simulink model "etc"  (R2022b)
settings: Solver=ode45  StartTime=0.0  StopTime=10.0  RelTol=1e-3  EnableMultiTasking=on
PreLoadFcn:
  | load busData;
  | load globData;
undefined symbols (not defined in the file): digital_range, direction_range_analog, duty_range_analog, Ts, uint_range_10bit
libraries: adcUtils x2, SignalEditorBlockLib x2
settings Model: Creator=jrivitus  LastModifiedBy=bensweet
settings SolverCC: MaxConsecutiveZCs=25  AlgebraicLoopSolver=TrustRegion
settings DataIOCC: LimitDataPoints=on  SaveFormat=Array  SaveOutput=off  SaveTime=off  ReturnWorkspaceOutputs=off
settings OptimizationCC: DefaultParameterBehavior=Inlined  ExpressionDepthLimit=2147483647  InitFltsAndDblsToZero=on  LifeSpan=inf
settings DebuggingCC: SolverPrmCheckMsg=warning  ParameterPrecisionLossMsg=none  FcnCallInpInsideContextMsg=warning  UnconnectedInputMsg=warning  UnconnectedOutputMsg=warning  UnconnectedLineMsg=warning  StateNameClashWarn=warning  PregeneratedLibrarySubsystemCodeDiagnostic=none  SFUnexpectedBacktrackingDiag=warning  SFNoUnconditionalDefaultTransitionDiag=warning  SFExecutionAtInitializationDiag=none  SFMachineParentedDataDiag=warning  ArithmeticOperatorsInVariantConditions=warning
settings HardwareCC: ProdBitPerPointer=32  ProdBitPerSizeT=32  ProdBitPerPtrDiffT=32  ProdLargestAtomicFloat=None  ProdIntDivRoundTo=Undefined  ProdEndianess=Unspecified  ProdWordSize=32  ProdHWDeviceType=32-bit Generic
settings ModelReferenceCC: EnableRefExpFcnMdlSchedulingChecks=on  PropagateSignalLabelsOutOfModel=off
settings SFSimCC: SimUseLocalCustomCode=off
settings RTWCC: RTWUseLocalCustomCode=off  DLArmComputeVersion=19.05
settings CodeAppCC: StateflowObjectComments=on
settings GRTTargetCC: TargetLangStandard=C89/C90 (ANSI)  CombineOutputUpdateFcns=off  GRTInterface=on
settings ConfigComp: CovMetricSettings=dw  CovSaveCumulativeToWorkspaceVar=on  CovSaveSingleToWorkspaceVar=on  CovExternalEMLEnable=off  CovSFcnEnable=off

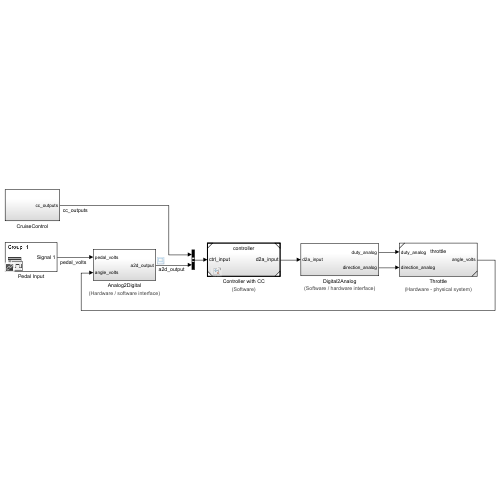
[thumbnail: Simulink's stored preview of the top-level diagram]
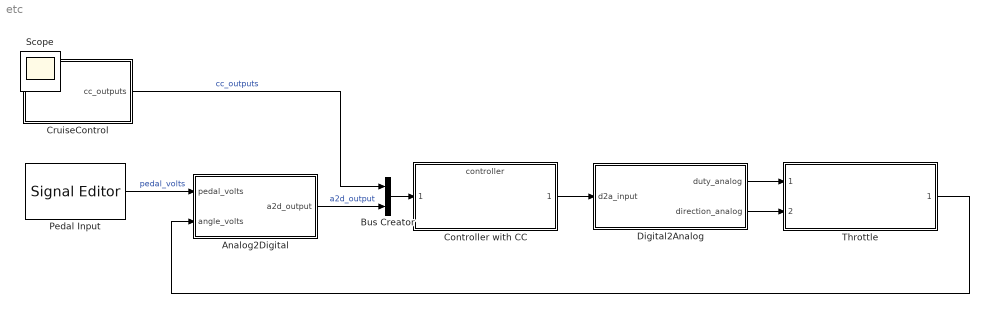
== system etc ==
  Analog2Digital : Subsystem
      settings: AttributesFormatString=(Hardware / software interface)  MinAlgLoopOccurrences=on
  Bus Creator : BusCreator  Inputs=2  OutDataTypeStr=Bus: ctrl_input_bus
  Controller with CC : ModelReference  ModelNameDialog=controller  SimulationMode=Normal  ModelReferenceVersion=6.0
      settings: AttributesFormatString=(Software)
  CruiseControl : Subsystem
      settings: MinAlgLoopOccurrences=on
  Digital2Analog : Subsystem
      settings: AttributesFormatString=(Software / hardware interface)  MinAlgLoopOccurrences=on
  Pedal Input : SignalEditorBlockLib/Signal Editor  FileName=etc_Pedal_Input.mat  ActiveScenario=Group_1  ActiveSignal=Signal 1  IsBus=off  OutputBusObjectStr=Bus: BusObject  SampleTime=0  OutputAfterFinalValue=Extrapolation  Unit=inherit  PreserveSignalName=on
  Throttle : Subsystem  ReferencedSubsystem=throttle
      settings: AttributesFormatString=(Hardware - physical system)
  Scope : Scope
  wires:
  Analog2Digital/1(a2d_output) -> Bus Creator/2  "a2d_output"
  CruiseControl/1(cc_outputs) -> Bus Creator/1  "cc_outputs"
  Digital2Analog/1(duty_analog) -> Throttle/1
  Digital2Analog/2(direction_analog) -> Throttle/2
  Throttle/1 -> Analog2Digital/2(angle_volts)
  Pedal Input/1 -> Analog2Digital/1(pedal_volts)  "pedal_volts"
  Bus Creator/1 -> Controller with CC/1
  Controller with CC/1 -> Digital2Analog/1(d2a_input)

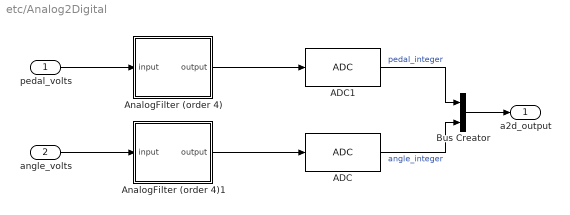
== system etc/Analog2Digital ==
  pedal_volts : Inport  OutDataTypeStr=double  PortDimensions=1  SampleTime=0
  angle_volts : Inport  Port=2  OutDataTypeStr=double  PortDimensions=1  SampleTime=0
  ADC : adcUtils/ADC  analog_range=angle_sensor_range  digital_range=uint_range_10bit  outputType=uint16  sampleTime=Ts
  ADC1 : adcUtils/ADC  analog_range=pedal_sensor_range  digital_range=uint_range_10bit  outputType=uint16  sampleTime=Ts
  AnalogFilter (order 4) : Subsystem  VariantControl=analogFilter==1
  AnalogFilter (order 4)1 : Subsystem  VariantControl=analogFilter==1
  Bus Creator : BusCreator  Inputs=2  OutDataTypeStr=Bus: a2d_output_bus
  a2d_output : Outport  OutDataTypeStr=Bus: a2d_output_bus  SampleTime=Ts  VectorParamsAs1DForOutWhenUnconnected=off
  wires:
  pedal_volts/1 -> AnalogFilter (order 4)/1(input)
  angle_volts/1 -> AnalogFilter (order 4)1/1(input)
  ADC1/1 -> Bus Creator/1  "pedal_integer"
  ADC/1 -> Bus Creator/2  "angle_integer"
  Bus Creator/1 -> a2d_output/1
  AnalogFilter (order 4)/1(output) -> ADC1/1
  AnalogFilter (order 4)1/1(output) -> ADC/1

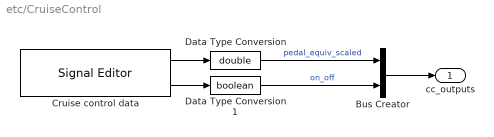
== system etc/CruiseControl ==
  Bus Creator : BusCreator  Inputs=2  OutDataTypeStr=Bus: cc_outputs_bus
  Cruise control data : SignalEditorBlockLib/Signal Editor  FileName=etc_CruiseControl_Cruise_control_data.mat  ActiveScenario=Group_1  ActiveSignal=on_off  IsBus=off  OutputBusObjectStr=Bus: BusObject  SampleTime=0  OutputAfterFinalValue=Extrapolation  Unit=inherit  PreserveSignalName=on
  Data Type Conversion : DataTypeConversion  OutDataTypeStr=double  SaturateOnIntegerOverflow=off  RndMeth=Floor
  Data Type Conversion1 : DataTypeConversion  OutDataTypeStr=boolean  SaturateOnIntegerOverflow=off  RndMeth=Floor
  cc_outputs : Outport  OutDataTypeStr=Bus: cc_outputs_bus  SampleTime=Ts  VectorParamsAs1DForOutWhenUnconnected=off
  wires:
  Cruise control data/1 -> Data Type Conversion/1
  Cruise control data/2 -> Data Type Conversion1/1
  Data Type Conversion/1 -> Bus Creator/1  "pedal_equiv_scaled"
  Data Type Conversion1/1 -> Bus Creator/2  "on_off"
  Bus Creator/1 -> cc_outputs/1

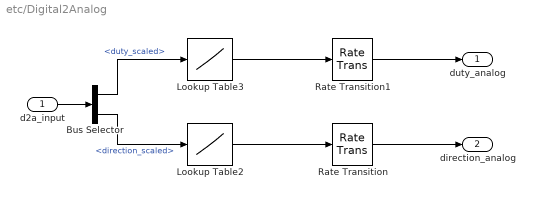
== system etc/Digital2Analog ==
  d2a_input : Inport  OutDataTypeStr=Bus: d2a_input_bus  PortDimensions=1  SampleTime=Ts
  Bus Selector : BusSelector  OutputSignals=duty_scaled,direction_scaled
  Lookup Table2 : Lookup_n-D  NumberOfTableDimensions=1  BreakpointsForDimension1=digital_range  Table=direction_range_analog  ExtrapMethod=Clip  OutDataTypeStr=double
      settings: AttributesFormatString=Output data type: %<OutDataTypeStr>
  Lookup Table3 : Lookup_n-D  NumberOfTableDimensions=1  BreakpointsForDimension1=uint_range_10bit  Table=duty_range_analog  ExtrapMethod=Clip  OutDataTypeStr=double
      settings: AttributesFormatString=Output data type: %<OutDataTypeStr>
  Rate Transition : RateTransition  Integrity=off  OutPortSampleTime=0
  Rate Transition1 : RateTransition  Integrity=off  OutPortSampleTime=0
  duty_analog : Outport  OutDataTypeStr=double  PortDimensions=1  SampleTime=0  VectorParamsAs1DForOutWhenUnconnected=off
  direction_analog : Outport  Port=2  OutDataTypeStr=double  PortDimensions=1  SampleTime=0  VectorParamsAs1DForOutWhenUnconnected=off
  wires:
  Bus Selector/2 -> Lookup Table2/1  "<direction_scaled>"
  Bus Selector/1 -> Lookup Table3/1  "<duty_scaled>"
  Rate Transition/1 -> direction_analog/1
  Rate Transition1/1 -> duty_analog/1
  Lookup Table3/1 -> Rate Transition1/1
  Lookup Table2/1 -> Rate Transition/1
  d2a_input/1 -> Bus Selector/1

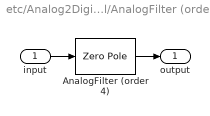
== system etc/Analog2Digital/AnalogFilter (order 4) ==
  input : Inport
  AnalogFilter (order 4) : ZeroPole  Zeros=[]  Poles=1.0e2*[-2.2739+0.6809i,-2.2739-0.6809i,-1.6518+2.0864i,-1.6518-2.0864i]  Gain=3.9899e9
  output : Outport  VectorParamsAs1DForOutWhenUnconnected=off
  wires:
  input/1 -> AnalogFilter (order 4)/1
  AnalogFilter (order 4)/1 -> output/1

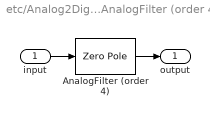
== system etc/Analog2Digital/AnalogFilter (order 4)1 ==
  input : Inport
  AnalogFilter (order 4) : ZeroPole  Zeros=[]  Poles=1.0e2*[-2.2739+0.6809i,-2.2739-0.6809i,-1.6518+2.0864i,-1.6518-2.0864i]  Gain=3.9899e9
  output : Outport  VectorParamsAs1DForOutWhenUnconnected=off
  wires:
  AnalogFilter (order 4)/1 -> output/1
  input/1 -> AnalogFilter (order 4)/1
